simulink model "BCU_tests"  (R2017b)
settings: Solver=FixedStepDiscrete  StartTime=0.0  StopTime=inf  FixedStep=Ts  RelTol=1e-3  EnableMultiTasking=on
settings Model: SimulationMode=external  Creator=OPPEL  LastModifiedBy=OPPEL
settings SolverCC: ConcurrentTasks=on  AutoInsertRateTranBlk=on
settings DataIOCC: SaveFormat=StructureWithTime
settings OptimizationCC: BlockReduction=off  OptimizeBlockIOStorage=off  BufferReuse=off  GlobalBufferReuse=off  ExpressionFolding=off  LocalBlockOutputs=off
settings HardwareCC: ProdBitPerPointer=32  ProdBitPerSizeT=32  ProdBitPerPtrDiffT=32  ProdLargestAtomicFloat=None  ProdWordSize=32  ProdLongLongMode=on  ProdHWDeviceType=Generic->32-bit x86 compatible
settings RTWCC: SystemTargetFile=slrt.tlc  TemplateMakefile=slrt_default_tmf  Description=Simulink Real-Time  CodeExecutionProfiling=on  RTWCompilerOptimization=on
settings CodeAppCC: StateflowObjectComments=on
settings SimulinkRealTimeCC: xPCisModelTimeout=off  xPCModelTimeoutSecs=20  xPCConcurrentTasks=on

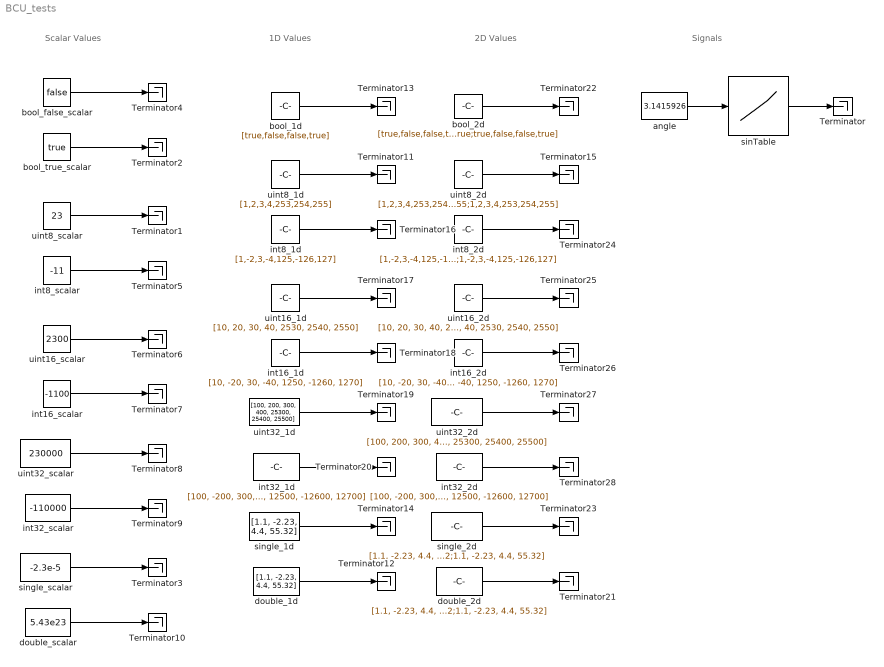
== system BCU_tests ==
  note: Scalar Values
  note: 1D Values
  note: 2D Values
  note: Signals
  Terminator{,1..28} (29 alike) : Terminator
  angle : Constant  Value=3.1415926  OutDataTypeStr=double
  bool_1d : Constant  Value=[true,false,false,true]  OutDataTypeStr=boolean
  bool_2d : Constant  Value=[true,false,false,true;true,false,false,true]  VectorParams1D=off  OutDataTypeStr=boolean
  bool_false_scalar : Constant  Value=false  OutDataTypeStr=boolean
  bool_true_scalar : Constant  Value=true  OutDataTypeStr=boolean
  double_1d : Constant  Value=[1.1, -2.23, 4.4, 55.32]  OutDataTypeStr=double
  double_2d : Constant  Value=[1.1, -2.23, 4.4, 55.32;1.1, -2.23, 4.4, 55.32;1.1, -2.23, 4.4, 55.32]  VectorParams1D=off  OutDataTypeStr=double
  double_scalar : Constant  Value=5.43e23  OutDataTypeStr=double
  int16_1d : Constant  Value=[10, -20, 30, -40, 1250, -1260, 1270]  OutDataTypeStr=int16
  int16_2d : Constant  Value=[10, -20, 30, -40, 1250, -1260, 1270;10, -20, 30, -40, 1250, -1260, 1270;10, -20, 30, -40, 1250, -1260, 1270;10, -20, 30, -40, 1250, -1260, 1270]  VectorParams1D=off  OutDataTypeStr=int16
  int16_scalar : Constant  Value=-1100  OutDataTypeStr=int16
  int32_1d : Constant  Value=[100, -200, 300, -400, 12500, -12600, 12700]  OutDataTypeStr=int32
  int32_2d : Constant  Value=[100, -200, 300, -400, 12500, -12600, 12700;100, -200, 300, -400, 12500, -12600, 12700;100, -200, 300, -400, 12500, -12600, 12700;100, -200, 300, -400, 12500, -12600, 12700]  OutDataTypeStr=int32
  int32_scalar : Constant  Value=-110000  OutDataTypeStr=int32
  int8_1d : Constant  Value=[1,-2,3,-4,125,-126,127]  OutDataTypeStr=int8
  int8_2d : Constant  Value=[1,-2,3,-4,125,-126,127;1,-2,3,-4,125,-126,127;1,-2,3,-4,125,-126,127;1,-2,3,-4,125,-126,127]  VectorParams1D=off  OutDataTypeStr=int8
  int8_scalar : Constant  Value=-11  OutDataTypeStr=int8
  sinTable : Lookup_n-D  NumberOfTableDimensions=1  BreakpointsForDimension1=[-5:5]  Table=tanh([-5:5])  TableDataTypeStr=Inherit: Inherit from 'Table data'  InternalRulePriority=Speed  RndMeth=Simplest  InputSameDT=on
  single_1d : Constant  Value=[1.1, -2.23, 4.4, 55.32]  OutDataTypeStr=single
  single_2d : Constant  Value=[1.1, -2.23, 4.4, 55.32;1.1, -2.23, 4.4, 55.32;1.1, -2.23, 4.4, 55.32]  VectorParams1D=off  OutDataTypeStr=single
  single_scalar : Constant  Value=-2.3e-5  OutDataTypeStr=single
  uint16_1d : Constant  Value=[10, 20, 30, 40, 2530, 2540, 2550]  OutDataTypeStr=uint16
  uint16_2d : Constant  Value=[10, 20, 30, 40, 2530, 2540, 2550;10, 20, 30, 40, 2530, 2540, 2550;10, 20, 30, 40, 2530, 2540, 2550;10, 20, 30, 40, 2530, 2540, 2550]  VectorParams1D=off  OutDataTypeStr=uint16
  uint16_scalar : Constant  Value=2300  OutDataTypeStr=uint16
  uint32_1d : Constant  Value=[100, 200, 300, 400, 25300, 25400, 25500]  OutDataTypeStr=uint32
  uint32_2d : Constant  Value=[100, 200, 300, 400, 25300, 25400, 25500;100, 200, 300, 400, 25300, 25400, 25500;100, 200, 300, 400, 25300, 25400, 25500;100, 200, 300, 400, 25300, 25400, 25500]  OutDataTypeStr=uint32
  uint32_scalar : Constant  Value=230000  OutDataTypeStr=uint32
  uint8_1d : Constant  Value=[1,2,3,4,253,254,255]  OutDataTypeStr=uint8
  uint8_2d : Constant  Value=[1,2,3,4,253,254,255;1,2,3,4,253,254,255;1,2,3,4,253,254,255;1,2,3,4,253,254,255]  VectorParams1D=off  OutDataTypeStr=uint8
  uint8_scalar : Constant  Value=23  OutDataTypeStr=uint8
  wires:
  uint8_scalar/1 -> Terminator1/1
  bool_true_scalar/1 -> Terminator2/1
  bool_false_scalar/1 -> Terminator4/1
  int8_scalar/1 -> Terminator5/1
  int16_scalar/1 -> Terminator7/1
  uint16_scalar/1 -> Terminator6/1
  uint32_scalar/1 -> Terminator8/1
  int32_scalar/1 -> Terminator9/1
  double_scalar/1 -> Terminator10/1
  single_scalar/1 -> Terminator3/1
  single_1d/1 -> Terminator14/1
  double_1d/1 -> Terminator12/1
  int32_1d/1 -> Terminator20/1
  uint32_1d/1 -> Terminator19/1
  uint16_1d/1 -> Terminator17/1
  int16_1d/1 -> Terminator18/1
  int8_1d/1 -> Terminator16/1
  bool_1d/1 -> Terminator13/1
  uint8_1d/1 -> Terminator11/1
  uint8_2d/1 -> Terminator15/1
  bool_2d/1 -> Terminator22/1
  int8_2d/1 -> Terminator24/1
  int16_2d/1 -> Terminator26/1
  uint16_2d/1 -> Terminator25/1
  uint32_2d/1 -> Terminator27/1
  int32_2d/1 -> Terminator28/1
  double_2d/1 -> Terminator21/1
  single_2d/1 -> Terminator23/1
  angle/1 -> sinTable/1
  sinTable/1 -> Terminator/1
